simulink subsystem "Mk3SerialTransmission"  (R2024b)
settings: Solver=VariableStepAuto  StartTime=0.0  StopTime=10.0  RelTol=1e-3
undefined symbols (not defined in the file): Motor1, Motor2, Motor3, Transmission1_Stage1, Transmission2_Stage1, Transmission3_Stage1
libraries: ssc_components x3
settings Model: DataDictionary=neck_mk3.sldd  EnableAccessToBaseWorkspace=off  Creator=upattacini  LastModifiedBy=upattacini
settings RTWCC: GPUComputeCapability=3.5

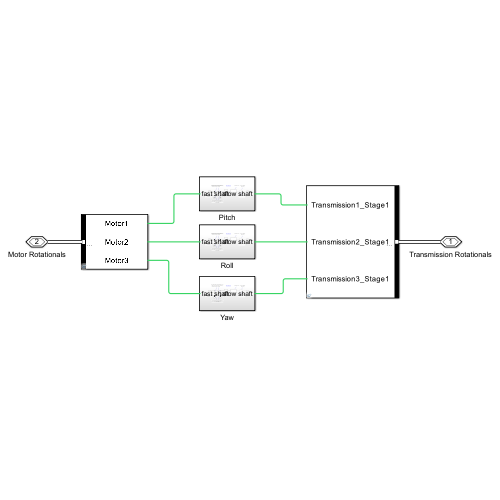
[thumbnail: Simulink's stored preview of the top-level diagram]
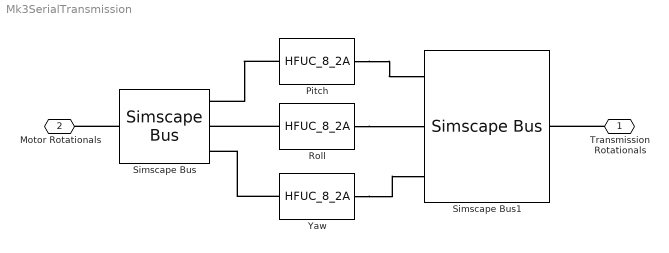
== system Mk3SerialTransmission ==
  Pitch : ssc_components/Transmissions/Harmonic Drives/HFUC_8_2A  SystemSampleTime=-1  VariantActivationTime=update diagram  AllowFlexibleInterface=on  Latency=0  AutoFrameSizeCalculation=off
  Roll : ssc_components/Transmissions/Harmonic Drives/HFUC_8_2A  SystemSampleTime=-1  VariantActivationTime=update diagram  AllowFlexibleInterface=on  Latency=0  AutoFrameSizeCalculation=off
  Simscape Bus : SimscapeBus  HierarchyStrings=Motor1;Motor2;Motor3  ConnectionType=Bus: Physical_MotorRotationals
  Simscape Bus1 : SimscapeBus  HierarchyStrings=Transmission1_Stage1;Transmission2_Stage1;Transmission3_Stage1  ConnectionType=Bus: Physical_TransmissionRotationals
  Yaw : ssc_components/Transmissions/Harmonic Drives/HFUC_8_2A  SystemSampleTime=-1  VariantActivationTime=update diagram  AllowFlexibleInterface=on  Latency=0  AutoFrameSizeCalculation=off
  Transmission Rotationals : PMIOPort  Side=Right  ConnectionType=Bus: Physical_TransmissionRotationals
  Motor Rotationals : PMIOPort  Port=2  Side=Left  ConnectionType=Bus: Physical_MotorRotationals
  connections:
  Simscape Bus/RConn1 -- Motor Rotationals/RConn1
  Yaw/LConn1 -- Simscape Bus/LConn3
  Pitch/LConn1 -- Simscape Bus/LConn1
  Roll/LConn1 -- Simscape Bus/LConn2
  Pitch/RConn1 -- Simscape Bus1/LConn1
  Roll/RConn1 -- Simscape Bus1/LConn2
  Yaw/RConn1 -- Simscape Bus1/LConn3
  Transmission Rotationals/RConn1 -- Simscape Bus1/RConn1
